simulink model "RI_PMSM_PI_PI"  (R2013b)
settings: Solver=ode45  StartTime=0.0  StopTime=10e-3  MaxStep=tau_d/50  RelTol=1e-3
InitFcn:
  | % Modellparaméterek
  | R = 440e-3;
  | L_dd = 155e-6;
  | L_qq = 188e-6;
  | 
  | Psi_PM = 24.5e-3;
  | z_P = 2;
  | 
  | J = 200e-7;
  | B = 5e-5;
  | 
  | 
  | % Rendszerparaméterek
  | K_d = 1/R;
  | tau_d = L_dd/R;
  | K_q = 1/R;
  | tau_q = L_qq/R;
  | 
  | K_M = 3/2*z_P*Psi_PM/B;
  | tau_M = J/B;
  | 
  | 
  | % Szabályzóhangolás
  | % Másodrendű zárt körként hangolva
  | 
  | % D-irányú áramkör
  | % i_dREF (= 0 A) -> u_d
  | xi_CL_d = 1;
  | tau_CL_d = tau_d/10;
  | 
  | K_PI_d_MRZK = (2*xi_CL_d*tau_d - tau_CL_d)/(K_d*tau_CL_d);
  | T_I_d_MRZK = (2*xi_CL_d*tau_d - tau_CL_d)*tau_CL_d/tau_d;
  | 
  | % Q-irányú áramkör
  | % i_qREF -> u_q
  | xi_CL_q = 1;
  | tau_CL_q = tau_q/10;
  | 
  | K_PI_q_MRZK = (2*xi_CL_q*tau_q - tau_CL_q)/(K_q*tau_CL_q);
  | T_I_q_MRZK = (2*xi_CL_q*tau_q - tau_CL_q)*tau_CL_q/tau_q;
  | 
  | % Forgó részrendszer
  | % omega_MREF -> i_qREF
  | xi_CL_M = 1;
  | tau_CL_M = tau_M/1000;
  | 
  | K_PI_M_MRZK = (2*xi_CL_M*tau_M - tau_CL_M)/(K_M*tau_CL_M);
  | T_I_M_MRZK = (2*xi_CL_M*tau_M - tau_CL_M)*tau_CL_M/tau_M;
libraries: RI_MK x6
settings Model: Creator=Szalay  LastModifiedBy=Szalay

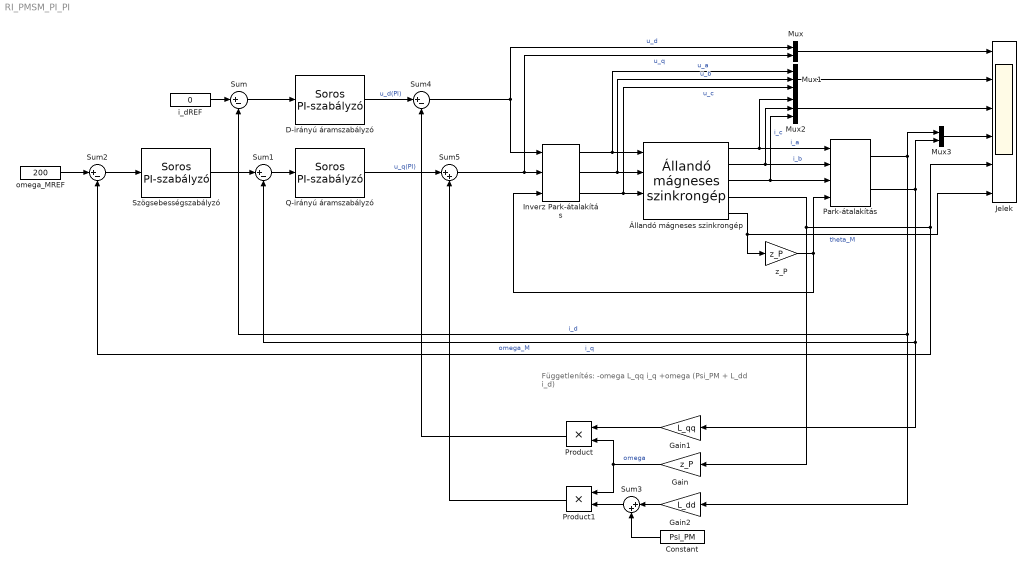
== system RI_PMSM_PI_PI ==
  note: Függetlenítés:
      | -omega L_qq i_q
      | +omega (Psi_PM + L_dd i_d)
  Constant : Constant  Value=Psi_PM
  D-irányú áramszabályzó : RI_MK/Soros PI-szabályzó  K_PI=K_PI_d_MRZK  T_I=T_I_d_MRZK
  Gain : Gain  Gain=z_P
  Gain1 : Gain  Gain=L_qq
  Gain2 : Gain  Gain=L_dd
  Inverz Park-átalakítás : RI_MK/Inverz Park-átalakítás
  Jelek : Scope  NumInputPorts=6
      settings: ShowLegends=on  YMin=-5~-5~-5~-5~-5~-5  YMax=5~5~5~5~5~5
  Mux : Mux  Inputs=2
  Mux1 : Mux  Inputs=3
  Mux2 : Mux  Inputs=3
  Mux3 : Mux  Inputs=2
  Park-átalakítás : RI_MK/Park-átalakítás
  Product : Product
  Product1 : Product
  Q-irányú áramszabályzó : RI_MK/Soros PI-szabályzó  K_PI=K_PI_q_MRZK  T_I=T_I_q_MRZK
  Sum{,1..2,4} (4 alike) : Sum  Inputs=|+-
  Sum3 : Sum  Inputs=|++
  Sum5 : Sum  Inputs=|++
  Szögsebességszabályzó : RI_MK/Soros PI-szabályzó  K_PI=K_PI_M_MRZK  T_I=T_I_M_MRZK
  i_dREF : Constant  Value=0
  omega_MREF : Constant  Value=200
  z_P : Gain  Gain=z_P
  Állandó mágneses szinkrongép : RI_MK/Állandó mágneses szinkrongép  R=R  L_dd=L_dd  L_qq=L_qq  Psi_PM=Psi_PM  z_P=z_P  J=J  B=B  i_d0=0  i_q0=0  omega_M0=0  theta_M0=0
  wires:
  Inverz Park-átalakítás/1 -> Mux1/1, Állandó mágneses szinkrongép/1  "u_a"
  Inverz Park-átalakítás/2 -> Mux1/2, Állandó mágneses szinkrongép/2  "u_b"
  Inverz Park-átalakítás/3 -> Mux1/3, Állandó mágneses szinkrongép/3  "u_c"
  Sum5/1 -> Mux/2, Inverz Park-átalakítás/2  "u_q"
  Állandó mágneses szinkrongép/5 -> Jelek/6, z_P/1  "theta_M"
  z_P/1 -> Inverz Park-átalakítás/3, Park-átalakítás/4
  Sum4/1 -> Mux/1, Inverz Park-átalakítás/1  "u_d"
  Mux/1 -> Jelek/1
  Mux1/1 -> Jelek/2
  Állandó mágneses szinkrongép/1 -> Park-átalakítás/1, Mux2/1  "i_a"
  Állandó mágneses szinkrongép/2 -> Park-átalakítás/2, Mux2/2  "i_b"
  Állandó mágneses szinkrongép/3 -> Park-átalakítás/3, Mux2/3  "i_c"
  Mux2/1 -> Jelek/3
  Park-átalakítás/1 -> Mux3/1, Gain2/1, Sum/2  "i_d"
  Park-átalakítás/2 -> Mux3/2, Gain1/1, Sum1/2  "i_q"
  Mux3/1 -> Jelek/4
  Állandó mágneses szinkrongép/4 -> Gain/1, Jelek/5, Sum2/2  "omega_M"
  Sum/1 -> D-irányú áramszabályzó/1
  Sum1/1 -> Q-irányú áramszabályzó/1
  Szögsebességszabályzó/1 -> Sum1/1
  Sum2/1 -> Szögsebességszabályzó/1
  i_dREF/1 -> Sum/1
  omega_MREF/1 -> Sum2/1
  D-irányú áramszabályzó/1 -> Sum4/1  "u_d(PI)"
  Gain/1 -> Product1/1, Product/2  "omega"
  Gain1/1 -> Product/1
  Sum3/1 -> Product1/2
  Gain2/1 -> Sum3/1
  Constant/1 -> Sum3/2
  Q-irányú áramszabályzó/1 -> Sum5/1  "u_q(PI)"
  Product/1 -> Sum4/2
  Product1/1 -> Sum5/2
